simulink model "MasterCtrl"  (R2020a)
settings: Solver=FixedStepDiscrete  StartTime=0.0  StopTime=10.0  FixedStep=0.5  RelTol=1e-3  EnableMultiTasking=on
libraries: simulink x2
settings Model: SILPILModeSetting=veronly  ExtModeTrigDuration=2  Creator=Sajad  LastModifiedBy=alireza
settings OptimizationCC: DefaultParameterBehavior=Inlined  UseDivisionForNetSlopeComputation=on  GainParamInheritBuiltInType=on  UseFloatMulNetSlope=on  InlineInvariantSignals=on  EnhancedBackFolding=on  BooleansAsBitfields=on  PassReuseOutputArgsAs=Individual arguments  StateBitsets=on  DataBitsets=on  ZeroExternalMemoryAtStartup=off  ZeroInternalMemoryAtStartup=off  NoFixptDivByZeroProtection=on  EfficientFloat2IntCast=on  LifeSpan=1  MaxStackSize=64  OptimizeBlockOrder=speed  DifferentSizesBufferReuse=on  EfficientTunableParamExpr=on
settings DebuggingCC: ParameterTunabilityLossMsg=error
settings HardwareCC: ProdBitPerInt=16  ProdBitPerPointer=16  ProdBitPerSizeT=16  ProdBitPerPtrDiffT=16  ProdLargestAtomicFloat=None  ProdWordSize=8  ProdHWDeviceType=Atmel->AVR
settings SFSimCC: MATLABDynamicMemAlloc=off  CustomCodeUndefinedFunction=UseInterfaceOnly
settings RTWCC: SystemTargetFile=ert.tlc  HardwareBoard=Arduino Uno  TLCOptions=-aInlineSetEventsForThisBaseRateFcn=TLC_FALSE -aSuppressMultiTaskScheduler=TLC_FALSE -aRateBasedStepFcn=1  TemplateMakefile=ert_default_tmf  GenerateReport=on  Toolchain=Arduino AVR  BuildConfiguration=Faster Runs  IncludeHyperlinkInReport=on  LaunchReport=on  GenerateTraceInfo=on  GenerateTraceReport=on  GenerateTraceReportSl=on  GenerateTraceReportSf=on  GenerateTraceReportEml=on  GenerateWebview=on
settings CodeAppCC: ForceParamTrailComments=on  IgnoreCustomStorageClasses=off  OperatorAnnotations=on  SimulinkDataObjDesc=on  SFDataObjDesc=on  CustomSymbolStrGlobalVar=rt$N$M  CustomSymbolStrType=$N$M  CustomSymbolStrFcn=$N$M$F  CustomSymbolStrMacro=$N$M  InsertBlockDesc=on
settings ERTTargetCC: TargetLangStandard=C99 (ISO)  IncludeMdlTerminateFcn=off  CombineSignalStateStructs=on  SupportAbsoluteTime=off  PurelyIntegerCode=on  SupportComplex=off  SupportNonInlinedSFcns=on  ExtModeStaticAllocSize=250  InlinedParameterPlacement=NonHierarchical  RootIOFormat=Structure reference  ERTFilePackagingFormat=CompactWithDataFile
settings ConfigComp: CovEnable=on  RecordCoverage=on  CovModelRefEnable=on

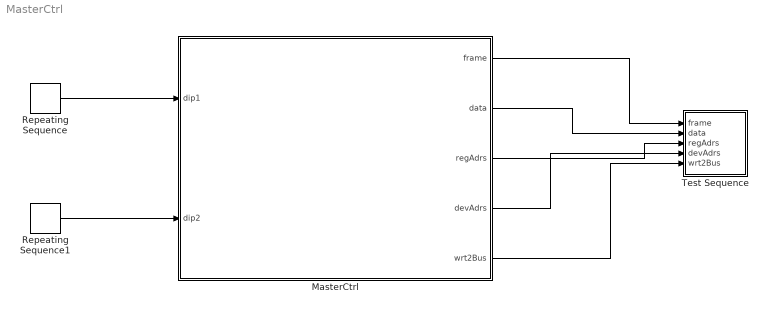
== system MasterCtrl ==
  MasterCtrl : Stateflow chart  TreatAsAtomicUnit=on
  Repeating Sequence : simulink/Sources/Repeating Sequence  rep_seq_t=[0 3 4 6 7 8 9]  rep_seq_y=[1 1 0 0 1 1 0]
  Repeating Sequence1 : simulink/Sources/Repeating Sequence  rep_seq_t=[0 3 4 7 8 9]  rep_seq_y=[0 0 1 1 1 0]
  Test Sequence : Test Sequence  TreatAsAtomicUnit=on
  wires:
  Repeating Sequence/1 -> MasterCtrl/1(dip1)
  Repeating Sequence1/1 -> MasterCtrl/2(dip2)
  MasterCtrl/1(frame) -> Test Sequence/1(frame)
  MasterCtrl/2(data) -> Test Sequence/2(data)
  MasterCtrl/3(regAdrs) -> Test Sequence/3(regAdrs)
  MasterCtrl/4(devAdrs) -> Test Sequence/4(devAdrs)
  MasterCtrl/5(wrt2Bus) -> Test Sequence/5(wrt2Bus)

== stateflow chart MasterCtrl/MasterCtrl ==
  state Read
    state Dip_1
      devAdrs = 2;
      regAdrs = -128;
      data = 0;
      wrt2Bus = 1;
    state Read_idle
    state Dip_2
      devAdrs = 3;
      regAdrs = -128;
      data = 0;
      wrt2Bus = 1;
    Read_idle -> Dip_1 [order 1] : [dip1 == 1]
    (default) -> Read_idle : { dip1; dip2 }
    Read_idle -> Dip_2 [order 2] : [dip2 == 1]
  state Write
    state Write_start
    state Device_Address
      frame = devAdrs
    state Register_Address
      frame = regAdrs
    state Data
      frame = data;
      wrt2Bus = 0;
    (default) -> Write_start
    Write_start -> Device_Address
    Device_Address -> Register_Address
    Register_Address -> Data
  (default) -> Read
  Write -> Read : [wrt2Bus == 0]
  Read -> Write : [wrt2Bus == 1]
  data: dip1 input double; dip2 input double; frame output int64; data output int64; regAdrs output int64; devAdrs output int64; wrt2Bus output double =0

== stateflow chart MasterCtrl/Test Sequence ==
  settings: stateMachineType=SIMPLIFIED_MACHINE
  state step_1
    assert(devAdrs==0 && regAdrs==0 && data==0)
  state step_2
    assert(devAdrs==2 && regAdrs==-128 && wrt2Bus==1)
  state step_3
    assert(frame==2 && devAdrs==2 && regAdrs==-128 && wrt2Bus==1)
  state step_4
    assert(frame==-128 && devAdrs==2 && regAdrs==-128 && wrt2Bus==1)
  state step_5
    assert(frame==0 && devAdrs==2 && regAdrs==-128 && wrt2Bus==0)
  state step_6
    assert(devAdrs==3 && regAdrs==-128 && wrt2Bus==1)
  state step_7
    assert(frame==3 && devAdrs==3 && regAdrs==-128 && wrt2Bus==1)
  state step_8
    assert(frame==-128 && devAdrs==3 && regAdrs==-128 && wrt2Bus==1)
  state step_9
    assert(frame==0 && devAdrs==3 && regAdrs==-128 && wrt2Bus==0)
  state step_10
  (default) -> step_1
  step_1 -> step_2 : [
      | after(0.5,sec)
      | ]
  step_2 -> step_3 : [
      | after(1,sec)
      | ]
  step_3 -> step_4 : [
      | after(0.5,sec)
      | ]
  step_4 -> step_5 : [
      | after(0.5,sec)
      | ]
  step_5 -> step_6 : [
      | after(1.5,sec)
      | ]
  step_6 -> step_7 : [
      | after(1,sec)
      | ]
  step_7 -> step_8 : [
      | after(0.5,sec)
      | ]
  step_8 -> step_9 : [
      | after(0.5,sec)
      | ]
  step_9 -> step_10 : [
      | after(0.5,sec)
      | ]
  data: frame input; data input; regAdrs input; devAdrs input; wrt2Bus input
